simulink model "harness"  (R2020b)
settings: Solver=FixedStepAuto  StartTime=0.0  StopTime=2  FixedStep=0.000001  RelTol=1e-3
settings Model: Creator=GUO HUI  LastModifiedBy=GUO HUI

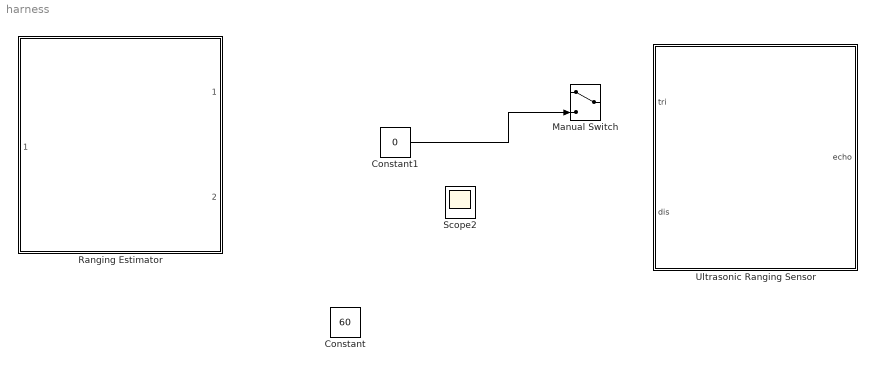
== system harness ==
  Constant : Constant  Value=60
  Constant1 : Constant  Value=0
  Manual Switch : ManualSwitch
  Ranging Estimator : Subsystem  TreatAsAtomicUnit=on  ReferencedSubsystem=Ranging_Estimator
  Scope2 : Scope
  Ultrasonic Ranging Sensor : Subsystem
  wires:
  Constant1/1 -> Manual Switch/2

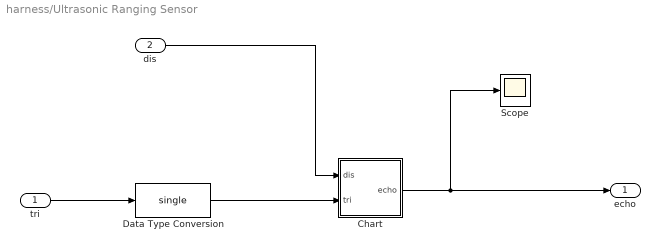
== system harness/Ultrasonic Ranging Sensor ==
  tri : Inport
  dis : Inport  Port=2
  Chart : Stateflow chart  TreatAsAtomicUnit=on
  Data Type Conversion : DataTypeConversion  OutDataTypeStr=single  LockScale=on
  Scope : Scope
  echo : Outport
  wires:
  tri/1 -> Data Type Conversion/1
  dis/1 -> Chart/1(dis)
  Chart/1(echo) -> Scope/1, echo/1
  Data Type Conversion/1 -> Chart/2(tri)

== stateflow chart harness/Ultrasonic Ranging Sensor/Chart ==
  state start
    en:echo=0
  state echo_up
    en:echo=1
    echodu=dis
  state echo_down
    en:echo=0
  echo_down -> start : [tri==0]
  (default) -> start
  echo_up -> echo_down : after(echodu*58,usec)
  start -> echo_up : [tri==1]
  data: dis input; tri input; echo output; echodu local
